simulink model "Phase_Shift_Keying"  (R2015a)
settings: Solver=ode3  StartTime=0.0  StopTime=10.0  FixedStep=0.01  RelTol=1e-3
settings Model: Creator=Chayti  LastModifiedBy=hp

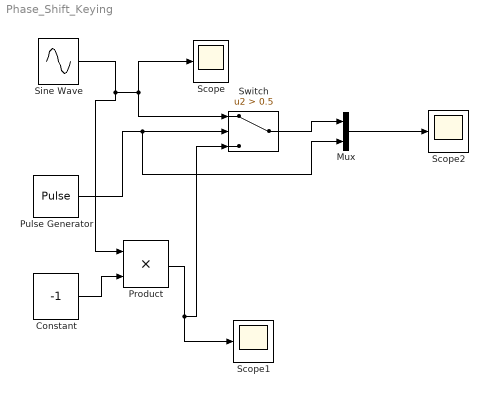
== system Phase_Shift_Keying ==
  Constant : Constant  Value=-1
  Mux : Mux  Inputs=2
  Product : Product
  Pulse Generator : DiscretePulseGenerator  PulseType=Time based  PulseWidth=50
  Scope : Scope
  Scope1 : Scope
  Scope2 : Scope
      settings: SaveName=ScopeData2
  Sine Wave : Sin  Frequency=2*pi*2  SampleTime=0.01
  Switch : Switch  Criteria=u2 > Threshold  Threshold=0.5
  wires:
  Sine Wave/1 -> Product/1, Scope/1, Switch/1
  Pulse Generator/1 -> Mux/2, Switch/2
  Constant/1 -> Product/2
  Product/1 -> Scope1/1, Switch/3
  Switch/1 -> Mux/1
  Mux/1 -> Scope2/1
